simulink model "Sim2"  (R2023a)
settings: Solver=FixedStepAuto  StartTime=0.0  StopTime=18  FixedStep=1e-4  RelTol=1e-3
values from neighbouring files (symbols this model uses):
  A1 = 28e-4    (= 0.0028)    [main.m]    (also in main2.m; main3.m; main4.m)
  a1 = 0.071e-4    (= 7.1e-06)    [main.m]    (also in main2.m; main3.m; main4.m)
  A2 = 32e-4    (= 0.0032)    [main.m]    (also in main2.m; main3.m; main4.m)
  a2 = 0.057e-4    (= 5.7e-06)    [main.m]    (also in main2.m; main3.m; main4.m)
  a3 = 0.071e-4    (= 7.1e-06)    [main.m]    (also in main2.m; main3.m; main4.m)
  A3 = 28e-4    (= 0.0028)    [main.m]    (also in main2.m; main3.m; main4.m)
  A4 = 32e-4    (= 0.0032)    [main.m]    (also in main2.m; main3.m; main4.m)
  a4 = 0.057e-4    (= 5.7e-06)    [main.m]    (also in main2.m; main3.m; main4.m)
  Com_H1 = 1.3*H01^2    [main.m]    (also in main2.m; main3.m; main4.m)
  Com_H2 = 1.3*H02^2    [main.m]    (also in main2.m; main3.m; main4.m)
  delay_Com_H1 = 2.5    [main.m]    (also in main2.m = 1.5; main3.m = 1.5; main4.m = 1.5)
  delay_Com_H2 = 1.5    [main.m]    (also in main2.m = 0.5; main3.m = 0.5; main4.m = 0.5)
  g = 9.81    [main.m]    (also in main2.m; main3.m; main4.m)
  gamma1 = 0.7    [main.m]    (also in main2.m; main3.m; main4.m)
  gamma2 = 0.6    [main.m]    (also in main2.m; main3.m; main4.m)
  H01 = (gamma1*k1*V01+(1-gamma2)*k2*V02)/(a1*sqrt(2*g))    [main.m]    (also in main2.m; main3.m; main4.m)
  H02 = (gamma2*k2*V02+(1-gamma1)*k1*V01)/(a2*sqrt(2*g))    [main.m]    (also in main2.m; main3.m; main4.m)
  H03 = (1-gamma2)*k2*V02/(a3*sqrt(2*g))    [main.m]    (also in main2.m; main3.m; main4.m)
  H04 = (1-gamma1)*k1*V01/(a4*sqrt(2*g))    [main.m]    (also in main2.m; main3.m; main4.m)
  k1 = 3.33e-6    (= 3.33e-06)    [main.m]    (also in main2.m; main3.m; main4.m)
  k2 = 3.35e-6    (= 3.35e-06)    [main.m]    (also in main2.m; main3.m; main4.m)
  kc1 = (2*xi*wo1*T1-1)/K11    [main.m]    (also in main2.m; main3.m; main4.m)
  kc2 = (2*xi*wo1*T2-1)/K22    [main.m]    (also in main2.m; main3.m; main4.m)
  Matrix_dX_U = [gamma1*k1/A1, 0 ... (first row only)    [main.m]    (also in main2.m; main3.m; main4.m)
  Matrix_dX_X = [-1/T1, 0, -A3/(A1*T3), 0 ... (first row only)    [main.m]    (also in main2.m; main3.m; main4.m)
  Matrix_H0 = [H01^2;H02^2;H03^2;H04^2]    [main.m]    (also in main2.m; main3.m; main4.m)
  Matrix_V0 = [V01;V02]    [main.m]    (also in main2.m; main3.m; main4.m)
  Tc1 = 2*xi/wo1-1/(T1*wo1^2)    [main.m]    (also in main2.m; main3.m; main4.m)
  Tc2 = 2*xi/wo2-1/(T2*wo2^2)    [main.m]    (also in main2.m; main3.m; main4.m)
libraries: slpidlib x4, simulink x2
settings Model: Creator=philippecasteres  LastModifiedBy=philippecasteres

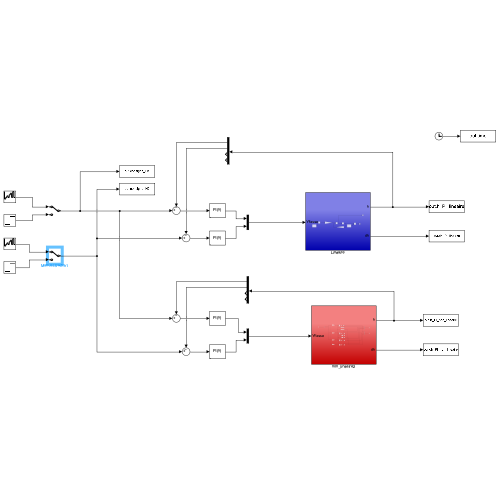
[thumbnail: Simulink's stored preview of the top-level diagram]
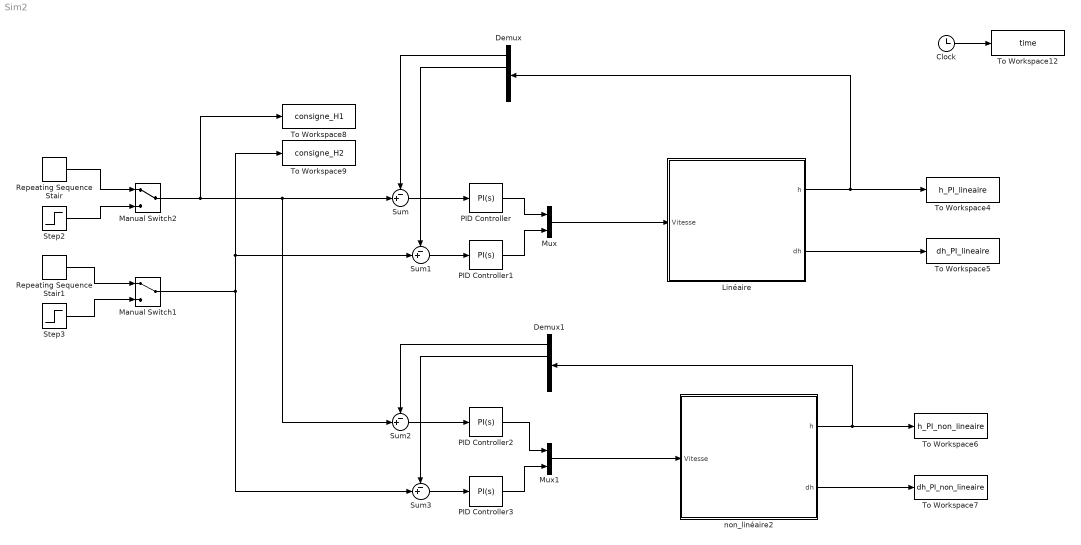
== system Sim2 ==
  Clock : Clock
  Demux : Demux
  Demux1 : Demux
  Linéaire : Subsystem
  Manual Switch1 : ManualSwitch
  Manual Switch2 : ManualSwitch
  Mux : Mux  Inputs=2
  Mux1 : Mux  Inputs=2
  PID Controller : slpidlib/PID Controller  Controller=PI  Form=Parallel  TimeDomain=Continuous-time  UseExternalTs=off  SampleTime=-1  IntegratorMethod=Forward Euler  FilterMethod=Forward Euler  ControllerParametersSource=internal  P=kc1  I=kc1/Tc1  UseKiTs=off  D=0  N=100  UseFilter=on  TunerSelectOption=Transfer Function Based (PID Tuner App)  InitialConditionSource=internal  InitialConditionForIntegrator=0  InitialConditionForFilter=0  DifferentiatorICPrevScaledInput=0  ExternalReset=none  TrackingMode=off  Kt=1  LimitOutput=off  SatLimitsSource=internal  UpperSaturationLimit=inf  LowerSaturationLimit=-inf  LinearizeAsGain=on  AntiWindupMode=none  Kb=1  LimitIntegrator=off  UpperIntegratorSaturationLimit=inf  LowerIntegratorSaturationLimit=-inf  POutMin=[]  POutMax=[]  IOutMin=[]  IOutMax=[]  DOutMin=[]  DOutMax=[]  NOutMin=[]  NOutMax=[]  SumOutMin=[]  SumOutMax=[]  SaturationOutMin=[]  SaturationOutMax=[]  PParamMin=[]  PParamMax=[]  IParamMin=[]  IParamMax=[]  DParamMin=[]  DParamMax=[]  NParamMin=[]  NParamMax=[]  KbParamMin=[]  KbParamMax=[]  KtParamMin=[]  KtParamMax=[]  KbOutMin=[]  KbOutMax=[]  KtOutMin=[]  KtOutMax=[]  IntegratorOutMin=[]  IntegratorOutMax=[]  FilterOutMin=[]  FilterOutMax=[]  SumI1OutMin=[]  SumI1OutMax=[]  SumI2OutMin=[]  SumI2OutMax=[]  SumI3OutMin=[]  SumI3OutMax=[]  SumI4OutMin=[]  SumI4OutMax=[]  SumDOutMin=[]  SumDOutMax=[]  DifferentiatorOutMin=[]  DifferentiatorOutMax=[]  FilterDiffOutCoefMin=[]  FilterDiffOutCoefMax=[]  ReciprocalOutMin=[]  ReciprocalOutMax=[]  SumDenOutMin=[]  SumDenOutMax=[]  SumNumOutMin=[]  SumNumOutMax=[]  DivideOutMin=[]  DivideOutMax=[]  UdiffTsProdOutMin=[]  UdiffTsProdOutMax=[]  NTsProdOutMin=[]  NTsProdOutMax=[]  UintegralTsProdOutMin=[]  UintegralTsProdOutMax=[]  UngainTsProdOutMin=[]  UngainTsProdOutMax=[]  ClampingZeroOutDataTypeStr=Inherit: Inherit via back propagation  ClampingZeroOutMin=[]  ClampingZeroOutMax=[]  FilterDenConstantOutDataTypeStr=Inherit: Inherit via back propagation  FilterDenConstantOutMin=[]  FilterDenConstantOutMax=[]  PCopyOutDataTypeStr=Inherit: Inherit via back propagation  PCopyOutMin=[]  PCopyOutMax=[]  NCopyOutDataTypeStr=Inherit: Inherit via back propagation  NCopyOutMin=[]  NCopyOutMax=[]  IntegratorContinuousStateAttributes=''  IntegratorStateMustResolveToSignalObject=off  IntegratorRTWStateStorageClass=Auto  FilterContinuousStateAttributes=''  FilterStateMustResolveToSignalObject=off  FilterRTWStateStorageClass=Auto  ParallelPVariant=InternalParameters  IdealPVariant=Disabled  IVariant=InternalParameters  DVariant=Disabled  IntegratorVariant=Continuous  SatVariant=Disabled  AWVariant=Passthrough  PCopyVariant=Disabled  TRVariant=Disabled  FdbkBlocksVariant=Forward  IdealPFdbkVariant=Disabled  SatFdbkVariant=Disabled  DerivativeFilterVariant=Disabled  NVariant=Disabled  NCopyVariant=Disabled_SignalSpec  FilterICVariant=Disabled  IntegratorICVariant=InternalICs  ExternalResetVariant=Disabled  TRSumVariant=Passthrough  SumFdbkVariant=Disabled  SumVariant=Sum_PI  TsampFilterVariant=InternalTs  TsampNgainVariant=Passthrough  TsampIntegralVariant=Disabled_SignalSpec  ExternalSaturationOutDataTypeStr=Inherit: Same as second input
  PID Controller1 : slpidlib/PID Controller  Controller=PI  Form=Parallel  TimeDomain=Continuous-time  UseExternalTs=off  SampleTime=-1  IntegratorMethod=Forward Euler  FilterMethod=Forward Euler  ControllerParametersSource=internal  P=kc2  I=kc2/Tc2  UseKiTs=off  D=0  N=100  UseFilter=on  TunerSelectOption=Transfer Function Based (PID Tuner App)  InitialConditionSource=internal  InitialConditionForIntegrator=0  InitialConditionForFilter=0  DifferentiatorICPrevScaledInput=0  ExternalReset=none  TrackingMode=off  Kt=1  LimitOutput=off  SatLimitsSource=internal  UpperSaturationLimit=inf  LowerSaturationLimit=-inf  LinearizeAsGain=on  AntiWindupMode=none  Kb=1  LimitIntegrator=off  UpperIntegratorSaturationLimit=inf  LowerIntegratorSaturationLimit=-inf  POutMin=[]  POutMax=[]  IOutMin=[]  IOutMax=[]  DOutMin=[]  DOutMax=[]  NOutMin=[]  NOutMax=[]  SumOutMin=[]  SumOutMax=[]  SaturationOutMin=[]  SaturationOutMax=[]  PParamMin=[]  PParamMax=[]  IParamMin=[]  IParamMax=[]  DParamMin=[]  DParamMax=[]  NParamMin=[]  NParamMax=[]  KbParamMin=[]  KbParamMax=[]  KtParamMin=[]  KtParamMax=[]  KbOutMin=[]  KbOutMax=[]  KtOutMin=[]  KtOutMax=[]  IntegratorOutMin=[]  IntegratorOutMax=[]  FilterOutMin=[]  FilterOutMax=[]  SumI1OutMin=[]  SumI1OutMax=[]  SumI2OutMin=[]  SumI2OutMax=[]  SumI3OutMin=[]  SumI3OutMax=[]  SumI4OutMin=[]  SumI4OutMax=[]  SumDOutMin=[]  SumDOutMax=[]  DifferentiatorOutMin=[]  DifferentiatorOutMax=[]  FilterDiffOutCoefMin=[]  FilterDiffOutCoefMax=[]  ReciprocalOutMin=[]  ReciprocalOutMax=[]  SumDenOutMin=[]  SumDenOutMax=[]  SumNumOutMin=[]  SumNumOutMax=[]  DivideOutMin=[]  DivideOutMax=[]  UdiffTsProdOutMin=[]  UdiffTsProdOutMax=[]  NTsProdOutMin=[]  NTsProdOutMax=[]  UintegralTsProdOutMin=[]  UintegralTsProdOutMax=[]  UngainTsProdOutMin=[]  UngainTsProdOutMax=[]  ClampingZeroOutDataTypeStr=Inherit: Inherit via back propagation  ClampingZeroOutMin=[]  ClampingZeroOutMax=[]  FilterDenConstantOutDataTypeStr=Inherit: Inherit via back propagation  FilterDenConstantOutMin=[]  FilterDenConstantOutMax=[]  PCopyOutDataTypeStr=Inherit: Inherit via back propagation  PCopyOutMin=[]  PCopyOutMax=[]  NCopyOutDataTypeStr=Inherit: Inherit via back propagation  NCopyOutMin=[]  NCopyOutMax=[]  IntegratorContinuousStateAttributes=''  IntegratorStateMustResolveToSignalObject=off  IntegratorRTWStateStorageClass=Auto  FilterContinuousStateAttributes=''  FilterStateMustResolveToSignalObject=off  FilterRTWStateStorageClass=Auto  ParallelPVariant=InternalParameters  IdealPVariant=Disabled  IVariant=InternalParameters  DVariant=Disabled  IntegratorVariant=Continuous  SatVariant=Disabled  AWVariant=Passthrough  PCopyVariant=Disabled  TRVariant=Disabled  FdbkBlocksVariant=Forward  IdealPFdbkVariant=Disabled  SatFdbkVariant=Disabled  DerivativeFilterVariant=Disabled  NVariant=Disabled  NCopyVariant=Disabled_SignalSpec  FilterICVariant=Disabled  IntegratorICVariant=InternalICs  ExternalResetVariant=Disabled  TRSumVariant=Passthrough  SumFdbkVariant=Disabled  SumVariant=Sum_PI  TsampFilterVariant=InternalTs  TsampNgainVariant=Passthrough  TsampIntegralVariant=Disabled_SignalSpec  ExternalSaturationOutDataTypeStr=Inherit: Same as second input
  PID Controller2 : slpidlib/PID Controller  Controller=PI  Form=Parallel  TimeDomain=Continuous-time  UseExternalTs=off  SampleTime=-1  IntegratorMethod=Forward Euler  FilterMethod=Forward Euler  ControllerParametersSource=internal  P=kc1  I=kc1/Tc1  UseKiTs=off  D=0  N=100  UseFilter=on  TunerSelectOption=Transfer Function Based (PID Tuner App)  InitialConditionSource=internal  InitialConditionForIntegrator=0  InitialConditionForFilter=0  DifferentiatorICPrevScaledInput=0  ExternalReset=none  TrackingMode=off  Kt=1  LimitOutput=off  SatLimitsSource=internal  UpperSaturationLimit=inf  LowerSaturationLimit=-inf  LinearizeAsGain=on  AntiWindupMode=none  Kb=1  LimitIntegrator=off  UpperIntegratorSaturationLimit=inf  LowerIntegratorSaturationLimit=-inf  POutMin=[]  POutMax=[]  IOutMin=[]  IOutMax=[]  DOutMin=[]  DOutMax=[]  NOutMin=[]  NOutMax=[]  SumOutMin=[]  SumOutMax=[]  SaturationOutMin=[]  SaturationOutMax=[]  PParamMin=[]  PParamMax=[]  IParamMin=[]  IParamMax=[]  DParamMin=[]  DParamMax=[]  NParamMin=[]  NParamMax=[]  KbParamMin=[]  KbParamMax=[]  KtParamMin=[]  KtParamMax=[]  KbOutMin=[]  KbOutMax=[]  KtOutMin=[]  KtOutMax=[]  IntegratorOutMin=[]  IntegratorOutMax=[]  FilterOutMin=[]  FilterOutMax=[]  SumI1OutMin=[]  SumI1OutMax=[]  SumI2OutMin=[]  SumI2OutMax=[]  SumI3OutMin=[]  SumI3OutMax=[]  SumI4OutMin=[]  SumI4OutMax=[]  SumDOutMin=[]  SumDOutMax=[]  DifferentiatorOutMin=[]  DifferentiatorOutMax=[]  FilterDiffOutCoefMin=[]  FilterDiffOutCoefMax=[]  ReciprocalOutMin=[]  ReciprocalOutMax=[]  SumDenOutMin=[]  SumDenOutMax=[]  SumNumOutMin=[]  SumNumOutMax=[]  DivideOutMin=[]  DivideOutMax=[]  UdiffTsProdOutMin=[]  UdiffTsProdOutMax=[]  NTsProdOutMin=[]  NTsProdOutMax=[]  UintegralTsProdOutMin=[]  UintegralTsProdOutMax=[]  UngainTsProdOutMin=[]  UngainTsProdOutMax=[]  ClampingZeroOutDataTypeStr=Inherit: Inherit via back propagation  ClampingZeroOutMin=[]  ClampingZeroOutMax=[]  FilterDenConstantOutDataTypeStr=Inherit: Inherit via back propagation  FilterDenConstantOutMin=[]  FilterDenConstantOutMax=[]  PCopyOutDataTypeStr=Inherit: Inherit via back propagation  PCopyOutMin=[]  PCopyOutMax=[]  NCopyOutDataTypeStr=Inherit: Inherit via back propagation  NCopyOutMin=[]  NCopyOutMax=[]  IntegratorContinuousStateAttributes=''  IntegratorStateMustResolveToSignalObject=off  IntegratorRTWStateStorageClass=Auto  FilterContinuousStateAttributes=''  FilterStateMustResolveToSignalObject=off  FilterRTWStateStorageClass=Auto  ParallelPVariant=InternalParameters  IdealPVariant=Disabled  IVariant=InternalParameters  DVariant=Disabled  IntegratorVariant=Continuous  SatVariant=Disabled  AWVariant=Passthrough  PCopyVariant=Disabled  TRVariant=Disabled  FdbkBlocksVariant=Forward  IdealPFdbkVariant=Disabled  SatFdbkVariant=Disabled  DerivativeFilterVariant=Disabled  NVariant=Disabled  NCopyVariant=Disabled_SignalSpec  FilterICVariant=Disabled  IntegratorICVariant=InternalICs  ExternalResetVariant=Disabled  TRSumVariant=Passthrough  SumFdbkVariant=Disabled  SumVariant=Sum_PI  TsampFilterVariant=InternalTs  TsampNgainVariant=Passthrough  TsampIntegralVariant=Disabled_SignalSpec  ExternalSaturationOutDataTypeStr=Inherit: Same as second input
  PID Controller3 : slpidlib/PID Controller  Controller=PI  Form=Parallel  TimeDomain=Continuous-time  UseExternalTs=off  SampleTime=-1  IntegratorMethod=Forward Euler  FilterMethod=Forward Euler  ControllerParametersSource=internal  P=kc2  I=kc2/Tc2  UseKiTs=off  D=0  N=100  UseFilter=on  TunerSelectOption=Transfer Function Based (PID Tuner App)  InitialConditionSource=internal  InitialConditionForIntegrator=0  InitialConditionForFilter=0  DifferentiatorICPrevScaledInput=0  ExternalReset=none  TrackingMode=off  Kt=1  LimitOutput=off  SatLimitsSource=internal  UpperSaturationLimit=inf  LowerSaturationLimit=-inf  LinearizeAsGain=on  AntiWindupMode=none  Kb=1  LimitIntegrator=off  UpperIntegratorSaturationLimit=inf  LowerIntegratorSaturationLimit=-inf  POutMin=[]  POutMax=[]  IOutMin=[]  IOutMax=[]  DOutMin=[]  DOutMax=[]  NOutMin=[]  NOutMax=[]  SumOutMin=[]  SumOutMax=[]  SaturationOutMin=[]  SaturationOutMax=[]  PParamMin=[]  PParamMax=[]  IParamMin=[]  IParamMax=[]  DParamMin=[]  DParamMax=[]  NParamMin=[]  NParamMax=[]  KbParamMin=[]  KbParamMax=[]  KtParamMin=[]  KtParamMax=[]  KbOutMin=[]  KbOutMax=[]  KtOutMin=[]  KtOutMax=[]  IntegratorOutMin=[]  IntegratorOutMax=[]  FilterOutMin=[]  FilterOutMax=[]  SumI1OutMin=[]  SumI1OutMax=[]  SumI2OutMin=[]  SumI2OutMax=[]  SumI3OutMin=[]  SumI3OutMax=[]  SumI4OutMin=[]  SumI4OutMax=[]  SumDOutMin=[]  SumDOutMax=[]  DifferentiatorOutMin=[]  DifferentiatorOutMax=[]  FilterDiffOutCoefMin=[]  FilterDiffOutCoefMax=[]  ReciprocalOutMin=[]  ReciprocalOutMax=[]  SumDenOutMin=[]  SumDenOutMax=[]  SumNumOutMin=[]  SumNumOutMax=[]  DivideOutMin=[]  DivideOutMax=[]  UdiffTsProdOutMin=[]  UdiffTsProdOutMax=[]  NTsProdOutMin=[]  NTsProdOutMax=[]  UintegralTsProdOutMin=[]  UintegralTsProdOutMax=[]  UngainTsProdOutMin=[]  UngainTsProdOutMax=[]  ClampingZeroOutDataTypeStr=Inherit: Inherit via back propagation  ClampingZeroOutMin=[]  ClampingZeroOutMax=[]  FilterDenConstantOutDataTypeStr=Inherit: Inherit via back propagation  FilterDenConstantOutMin=[]  FilterDenConstantOutMax=[]  PCopyOutDataTypeStr=Inherit: Inherit via back propagation  PCopyOutMin=[]  PCopyOutMax=[]  NCopyOutDataTypeStr=Inherit: Inherit via back propagation  NCopyOutMin=[]  NCopyOutMax=[]  IntegratorContinuousStateAttributes=''  IntegratorStateMustResolveToSignalObject=off  IntegratorRTWStateStorageClass=Auto  FilterContinuousStateAttributes=''  FilterStateMustResolveToSignalObject=off  FilterRTWStateStorageClass=Auto  ParallelPVariant=InternalParameters  IdealPVariant=Disabled  IVariant=InternalParameters  DVariant=Disabled  IntegratorVariant=Continuous  SatVariant=Disabled  AWVariant=Passthrough  PCopyVariant=Disabled  TRVariant=Disabled  FdbkBlocksVariant=Forward  IdealPFdbkVariant=Disabled  SatFdbkVariant=Disabled  DerivativeFilterVariant=Disabled  NVariant=Disabled  NCopyVariant=Disabled_SignalSpec  FilterICVariant=Disabled  IntegratorICVariant=InternalICs  ExternalResetVariant=Disabled  TRSumVariant=Passthrough  SumFdbkVariant=Disabled  SumVariant=Sum_PI  TsampFilterVariant=InternalTs  TsampNgainVariant=Passthrough  TsampIntegralVariant=Disabled_SignalSpec  ExternalSaturationOutDataTypeStr=Inherit: Same as second input
  Repeating Sequence Stair : simulink/Sources/Repeating Sequence Stair  OutValues=Com_H1_sched  tsamp=T_plage  OutMin=[]  OutMax=[]  OutDataTypeStr=double  OutputDataTypeScalingMode=double  OutDataType=fixdt(0,8)  ConRadixGroup=Best Precision: Vector-wise  OutScaling=2^-12
  Repeating Sequence Stair1 : simulink/Sources/Repeating Sequence Stair  OutValues=Com_H2_sched  tsamp=T_plage  OutMin=[]  OutMax=[]  OutDataTypeStr=double  OutputDataTypeScalingMode=double  OutDataType=fixdt(0,8)  ConRadixGroup=Best Precision: Vector-wise  OutScaling=2^-12
  Step2 : Step  Time=delay_Com_H1  Before=H01^2  After=Com_H1  SampleTime=0
  Step3 : Step  Time=delay_Com_H2  Before=H02^2  After=Com_H2  SampleTime=0
  Sum{,1..3} (4 alike) : Sum  Inputs=-+|
  To Workspace12 : ToWorkspace  VariableName=time  SaveFormat=Timeseries  SampleTime=-1
  To Workspace4 : ToWorkspace  VariableName=h_PI_lineaire  SaveFormat=Timeseries  SampleTime=-1
  To Workspace5 : ToWorkspace  VariableName=dh_PI_lineaire  SaveFormat=Timeseries  SampleTime=-1
  To Workspace6 : ToWorkspace  VariableName=h_PI_non_lineaire  SaveFormat=Timeseries  SampleTime=-1
  To Workspace7 : ToWorkspace  VariableName=dh_PI_non_lineaire  SaveFormat=Timeseries  SampleTime=-1
  To Workspace8 : ToWorkspace  VariableName=consigne_H1  SaveFormat=Timeseries  SampleTime=-1
  To Workspace9 : ToWorkspace  VariableName=consigne_H2  SaveFormat=Timeseries  SampleTime=-1
  non_linéaire2 : Subsystem
  wires:
  Sum/1 -> PID Controller/1
  PID Controller1/1 -> Mux/2
  Sum2/1 -> PID Controller2/1
  Demux1/1 -> Sum2/1
  Linéaire/2(dh) -> To Workspace5/1
  Linéaire/1(h) -> To Workspace4/1, Demux/1
  PID Controller2/1 -> Mux1/1
  PID Controller3/1 -> Mux1/2
  Manual Switch1/1 -> To Workspace9/1, Sum1/2, Sum3/2
  Demux1/2 -> Sum3/1
  Mux/1 -> Linéaire/1(Vitesse)
  Demux/1 -> Sum/1
  Sum1/1 -> PID Controller1/1
  Repeating Sequence Stair/1 -> Manual Switch2/1
  PID Controller/1 -> Mux/1
  Manual Switch2/1 -> To Workspace8/1, Sum2/2, Sum/2
  non_linéaire2/2(dh) -> To Workspace7/1
  Sum3/1 -> PID Controller3/1
  Step2/1 -> Manual Switch2/2
  Demux/2 -> Sum1/1
  non_linéaire2/1(h) -> To Workspace6/1, Demux1/1
  Step3/1 -> Manual Switch1/2
  Mux1/1 -> non_linéaire2/1(Vitesse)
  Repeating Sequence Stair1/1 -> Manual Switch1/1
  Clock/1 -> To Workspace12/1

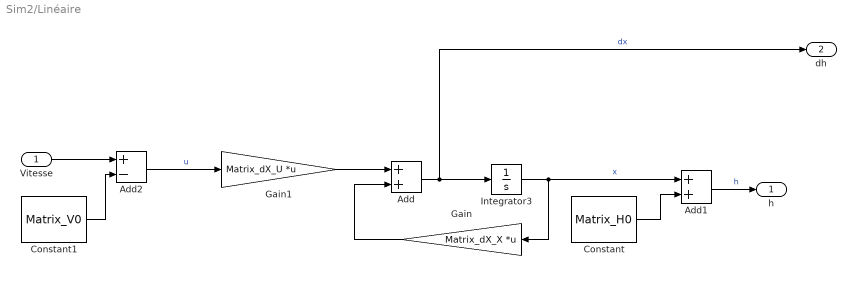
== system Sim2/Linéaire ==
  Vitesse : Inport
  Add : Sum
  Add1 : Sum
  Add2 : Sum  Inputs=+-
  Constant : Constant  Value=Matrix_H0
  Constant1 : Constant  Value=Matrix_V0
  Gain : Gain  Gain=Matrix_dX_X  Multiplication=Matrix(K*u)
  Gain1 : Gain  Gain=Matrix_dX_U  Multiplication=Matrix(K*u) (u vector)
  Integrator3 : Integrator
  h : Outport
  dh : Outport  Port=2
  wires:
  Constant/1 -> Add1/2
  Add1/1 -> h/1  "h"
  Add2/1 -> Gain1/1  "u"
  Vitesse/1 -> Add2/1
  Gain/1 -> Add/2
  Constant1/1 -> Add2/2
  Gain1/1 -> Add/1
  Add/1 -> Integrator3/1, dh/1  "dx"
  Integrator3/1 -> Add1/1, Gain/1  "x"

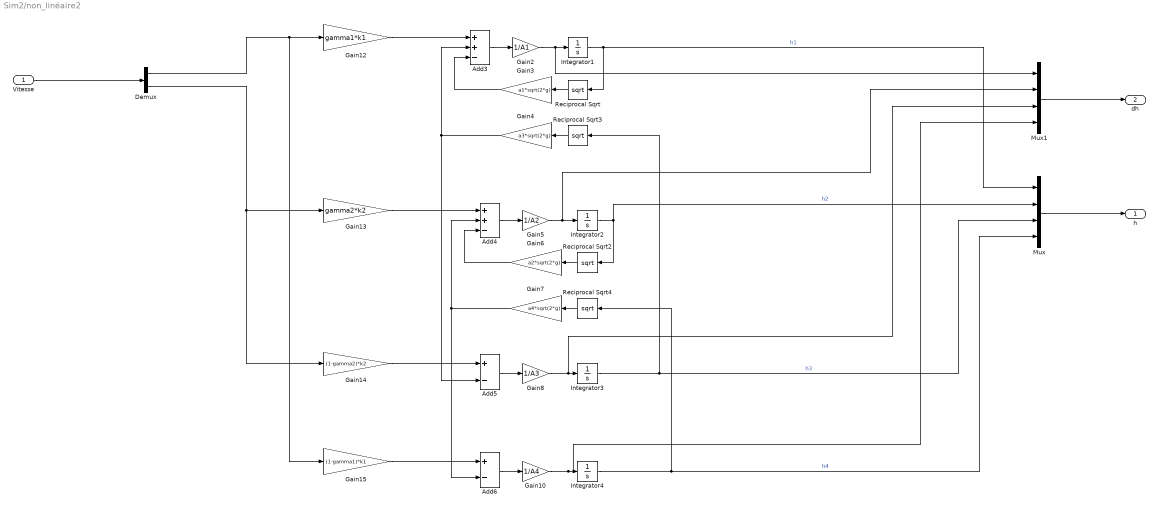
== system Sim2/non_linéaire2 ==
  Vitesse : Inport
  Add3 : Sum  Inputs=++-
  Add4 : Sum  Inputs=++-
  Add5 : Sum  Inputs=+-
  Add6 : Sum  Inputs=+-
  Demux : Demux  Outputs=2
  Gain10 : Gain  Gain=1/A4
  Gain12 : Gain  Gain=gamma1*k1
  Gain13 : Gain  Gain=gamma2*k2
  Gain14 : Gain  Gain=(1-gamma2)*k2
  Gain15 : Gain  Gain=(1-gamma1)*k1
  Gain2 : Gain  Gain=1/A1
  Gain3 : Gain  Gain=a1*sqrt(2*g)
  Gain4 : Gain  Gain=a3*sqrt(2*g)
  Gain5 : Gain  Gain=1/A2
  Gain6 : Gain  Gain=a2*sqrt(2*g)
  Gain7 : Gain  Gain=a4*sqrt(2*g)
  Gain8 : Gain  Gain=1/A3
  Integrator1 : Integrator  InitialCondition=H01^2
  Integrator2 : Integrator  InitialCondition=H02^2
  Integrator3 : Integrator  InitialCondition=H03^2
  Integrator4 : Integrator  InitialCondition=H04^2
  Mux : Mux
  Mux1 : Mux
  Reciprocal Sqrt{,2..4} (4 alike) : Sqrt
  h : Outport
  dh : Outport  Port=2
  wires:
  Add3/1 -> Gain2/1
  Gain2/1 -> Mux1/1, Integrator1/1
  Integrator1/1 -> Reciprocal Sqrt/1, Mux/1  "h1"
  Gain3/1 -> Add3/3
  Gain4/1 -> Add5/2, Add3/2
  Reciprocal Sqrt/1 -> Gain3/1
  Gain6/1 -> Add4/3
  Gain5/1 -> Mux1/2, Integrator2/1
  Add4/1 -> Gain5/1
  Integrator2/1 -> Mux/2, Reciprocal Sqrt2/1  "h2"
  Reciprocal Sqrt2/1 -> Gain6/1
  Gain7/1 -> Add6/2, Add4/2
  Add5/1 -> Gain8/1
  Reciprocal Sqrt3/1 -> Gain4/1
  Gain8/1 -> Mux1/3, Integrator3/1
  Integrator3/1 -> Mux/3, Reciprocal Sqrt3/1  "h3"
  Reciprocal Sqrt4/1 -> Gain7/1
  Integrator4/1 -> Mux/4, Reciprocal Sqrt4/1  "h4"
  Gain10/1 -> Mux1/4, Integrator4/1
  Add6/1 -> Gain10/1
  Mux/1 -> h/1
  Mux1/1 -> dh/1
  Gain12/1 -> Add3/1
  Gain13/1 -> Add4/1
  Gain15/1 -> Add6/1
  Gain14/1 -> Add5/1
  Demux/1 -> Gain15/1, Gain12/1
  Demux/2 -> Gain14/1, Gain13/1
  Vitesse/1 -> Demux/1
